simulink model "manipulator"  (R2021b)
settings: Solver=VariableStepAuto  StartTime=0.0  StopTime=10  RelTol=1e-3
InitFcn:
  | K=0.1;
  | 
  | m=10;
  | g=9.81;
  | d = 0.5;
  | 
  | J1 = 1;
  | J2 = 10;
settings Model: Creator=szmis  LastModifiedBy=szmis

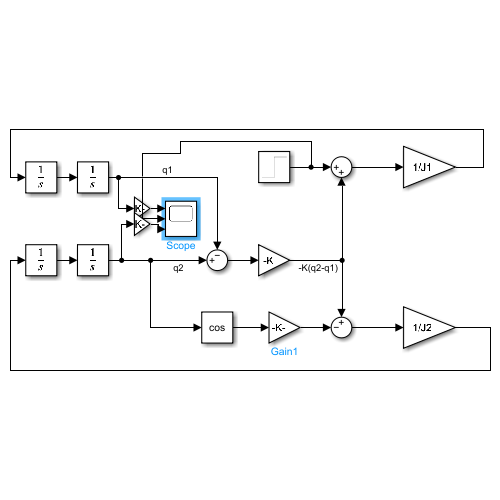
[thumbnail: Simulink's stored preview of the top-level diagram]
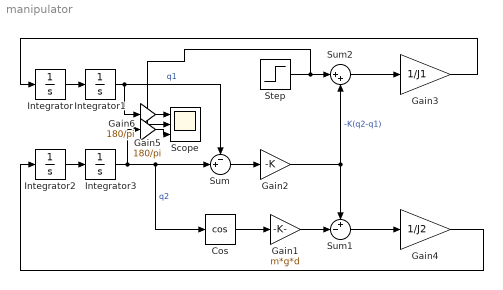
== system manipulator ==
  Cos : Trigonometry  Operator=cos
  Gain1 : Gain  Gain=m*g*d
  Gain2 : Gain  Gain=-K
  Gain3 : Gain  Gain=1/J1
  Gain4 : Gain  Gain=1/J2
  Gain5 : Gain  Gain=180/pi
  Gain6 : Gain  Gain=180/pi
  Integrator{,1..3} (4 alike) : Integrator
  Scope : Scope  NumInputPorts=3
  Step : Step  Time=2  After=2  SampleTime=0
  Sum : Sum  Inputs=-+|
  Sum1 : Sum  Inputs=+-|
  Sum2 : Sum  Inputs=|++
  wires:
  Cos/1 -> Gain1/1
  Gain4/1 -> Integrator2/1
  Sum/1 -> Gain2/1
  Gain2/1 -> Sum2/2, Sum1/1  "-K(q2-q1)"
  Gain1/1 -> Sum1/2
  Step/1 -> Scope/2, Sum2/1
  Sum2/1 -> Gain3/1
  Sum1/1 -> Gain4/1
  Gain3/1 -> Integrator/1
  Integrator1/1 -> Gain5/1, Sum/1  "q1"
  Integrator/1 -> Integrator1/1
  Integrator2/1 -> Integrator3/1
  Integrator3/1 -> Cos/1, Sum/2, Gain6/1  "q2"
  Gain5/1 -> Scope/1
  Gain6/1 -> Scope/3
